simulink model "WDS_MHE"  (R2022a)
settings: Solver=FixedStepDiscrete  StartTime=0.0  StopTime=T_final  FixedStep=T_sample  RelTol=1e-3
values from neighbouring files (symbols this model uses):
  A1 = inv(S1)*IO*U_i.'    [Run_model.m]
  A2 = OI*U_i.'    [Run_model.m]
  A_bar_d = readmatrix('A_bar_d.csv')    [Run_model.m]    (also in prepare_trajectory_data.m = [0.9950 0.0998)
  A_in1 = [zeros(size(HL_u,1),T*n_states), HL_u ... (first row only)    [Run_model.m]
  A_in2 = [zeros(size(HL_u,1),n_meas*T) ... (first row only)    [Run_model.m]
  b1p = inv(S1)*IO*U_history.'    [Run_model.m]
  b2p = OI*U_history.'    [Run_model.m]
  B_bar_d = readmatrix('B_bar_d.csv')    [Run_model.m]    (also in prepare_trajectory_data.m = [0.1)
  BDD_thresh = 5    [Run_model.m]
  C_obsv_d = [-0.48244804282  -0.463279461508; 0.0144227342104  -0.230554726046; 0.244765695792  -0.329721244669; 0.487562807757  0.730038636795; 0.684075320502  -0.191202440855; 0.0380669049625  0.232348391545]    [C_obsv_d.mat]    (also in Run_model.m = readmatrix('C_obsv_d.csv'); sys_generation_WDS.m = C_obsv)
  CE_MH = kron(eye(T),C_E)    [Run_model.m]
  Cm = ones(1,n_states)    [Run_model.m]
  D_obsv_d = readmatrix('D_obsv_d.csv')    [Run_model.m]    (also in prepare_trajectory_data.m = zeros(n_meas,n_int); sys_generation_WDS.m = D_obsv)
  DE_MH = kron(eye(T),D_E)    [Run_model.m]
  e_ini_matrix = reshape(e_ini,n_meas,T)    [Run_model.m]
  E_MH = kron(eye(T),E)    [Run_model.m]
  I = sort(randperm(n_meas,n_attack)).'    [Run_model.m]
  I_attack_ini = repmat(I,1,T)    [Run_model.m]
  K = place(A_bar_d,B_bar_d,Pc)    [Run_model.m]
  max_iter = 5000    [Run_model.m]
  n_alpha = size(HL_u,2)    [Run_model.m]
  n_meas = size(C_obsv_d,1)    [Run_model.m]    (also in prepare_trajectory_data.m = 6; sys_generation_WDS.m = size(C_obsv,1); test.m = size(C,1))
  n_states = 10    [sys_generation_WDS.m]    (also in test.m = size(A,1))
  offset = -inv(B_bar_d)*(A_bar_d-eye(n_states))*xd    [Run_model.m]
  T = 2*n_states    [Run_model.m]    (also in prepare_trajectory_data.m = 5)
  T_sample = 0.01    [Run_model.m]    (also in plot_error_table.m; prepare_trajectory_data.m; sys_generation_WDS.m; test.m)
  T_start_attack = .2*T_final    (= 1.6)    [Run_model.m]
  T_start_opt = load('Results/Data3.mat').T_start_opt    [plot_error_table.m]
  U0 = zeros(n_int,T+1)    [Run_model.m]
  x0 = 0.3+ 0.2*rand(n_states,1)    [Run_model.m]    (also in prepare_trajectory_data.m = [7;7]; test.m = rand(n_states,1))
  xd = 0.5*ones(n_states,1)    [Run_model.m]
  Y0 = zeros(n_meas,T)    [Run_model.m]
libraries: simulink x3
settings Model: Creator=Abelb  LastModifiedBy=Abelb
settings DebuggingCC: UnconnectedInputMsg=warning  UnconnectedOutputMsg=warning  UnconnectedLineMsg=warning
settings RTWCC: DLArmComputeVersion=19.05

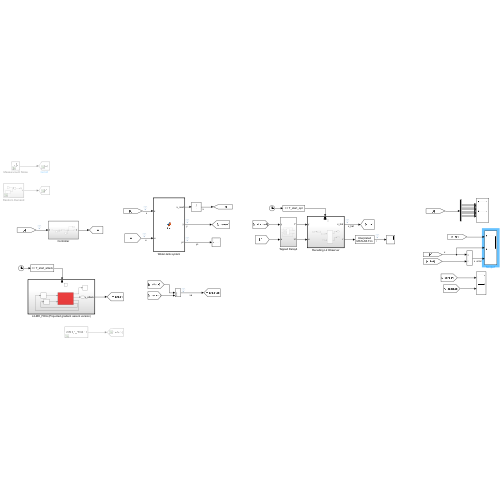
[thumbnail: Simulink's stored preview of the top-level diagram]
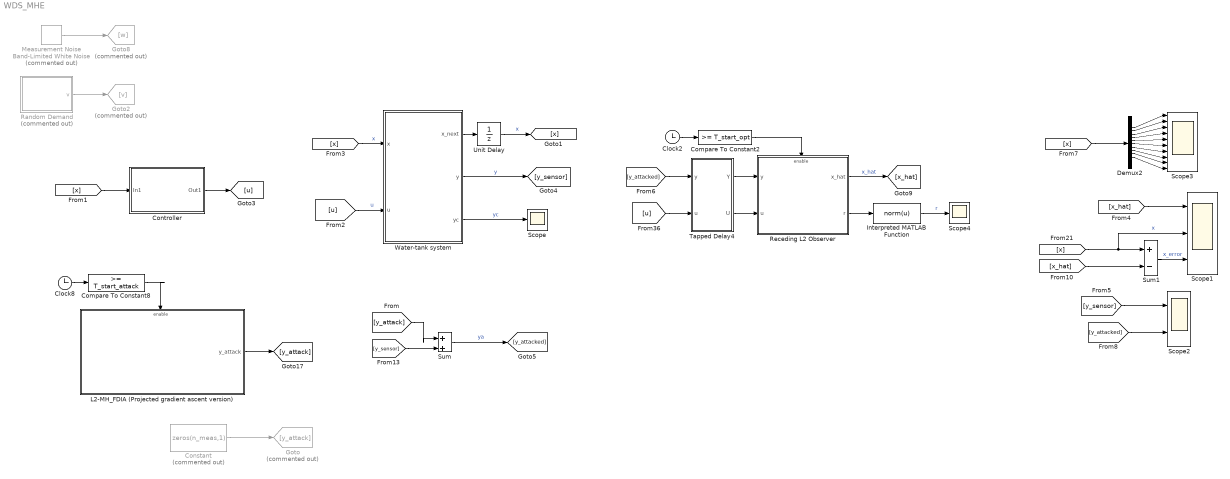
== system WDS_MHE ==
  Clock2 : Clock
  Clock8 : Clock
  Compare To Constant2 : simulink/Logic and Bit Operations/Compare To Constant  relop=>=  const=T_start_opt  OutDataTypeStr=boolean
  Compare To Constant8 : simulink/Logic and Bit Operations/Compare To Constant  relop=>=  const=T_start_attack  OutDataTypeStr=boolean
  Constant : Constant  Commented=on  Value=zeros(n_meas,1)
  Controller : Subsystem
  Demux2 : Demux  Outputs=n_states
  Goto : Goto  Commented=on  GotoTag=y_attack
  Goto2 : Goto  Commented=on  GotoTag=v
  Goto8 : Goto  Commented=on  GotoTag=w
  Interpreted MATLAB Function : MATLABFcn  MATLABFcn=norm(u)
  L2-MH_FDIA (Projected gradient ascent version) : Subsystem
  Measurement Noise : simulink/Sources/Band-Limited White Noise  Commented=on  Cov=[0.001]  Ts=T_sample  seed=[23341]
  Random Demand : Subsystem  Commented=on
  Receding L2 Observer : Subsystem
  Scope : Scope
  Scope1 : Scope  NumInputPorts=3
  Scope2 : Scope  NumInputPorts=2
  Scope3 : Scope  NumInputPorts=10
  Scope4 : Scope
  Sum : Sum  Inputs=|++
  Sum1 : Sum  Inputs=+-
  Tapped Delay4 : Subsystem
  Unit Delay : UnitDelay  InitialCondition=x0  SampleTime=-1  HasFrameUpgradeWarning=on
  Water-tank system : MATLAB Function  TreatAsAtomicUnit=on
  wires:
  Water-tank system/1(x_next) -> Unit Delay/1
  [u] -> Water-tank system/2(u)  "u"
  Tapped Delay4/2(U) -> Receding L2 Observer/2(u)
  Receding L2 Observer/1(x_hat) -> [x_hat]  "x_hat"
  [u] -> Tapped Delay4/2(u)
  Compare To Constant2/1 -> Receding L2 Observer/Enable
  Tapped Delay4/1(Y) -> Receding L2 Observer/1(y)
  Clock2/1 -> Compare To Constant2/1
  Demux2/4 -> Scope3/4
  Demux2/3 -> Scope3/3
  Demux2/5 -> Scope3/5
  Demux2/9 -> Scope3/9
  Demux2/10 -> Scope3/10
  Demux2/7 -> Scope3/7
  Demux2/1 -> Scope3/1
  Demux2/6 -> Scope3/6
  Demux2/2 -> Scope3/2
  Demux2/8 -> Scope3/8
  Interpreted MATLAB Function/1 -> Scope4/1  "r"
  Receding L2 Observer/2(r) -> Interpreted MATLAB Function/1
  [x] -> Controller/1(In1)
  Controller/1(Out1) -> [u]
  [x] -> Demux2/1
  Sum1/1 -> Scope1/3  "x_error"
  [x] -> Scope1/2, Sum1/1  "x"
  [x_hat] -> Sum1/2
  Water-tank system/3(yc) -> Scope/1  "yc"
  Unit Delay/1 -> [x]  "x"
  [x] -> Water-tank system/1(x)  "x"
  [x_hat] -> Scope1/1
  Compare To Constant8/1 -> L2-MH_FDIA (Projected gradient ascent version)/Enable
  Clock8/1 -> Compare To Constant8/1
  L2-MH_FDIA (Projected gradient ascent version)/1(y_attack) -> [y_attack]
  [y_sensor] -> Scope2/1
  [y_attacked] -> Tapped Delay4/1(y)
  Constant/1 -> Goto/1
  Measurement Noise/1 -> Goto8/1
  Random Demand/1(v) -> Goto2/1
  Water-tank system/2(y) -> [y_sensor]  "y"
  [y_sensor] -> Sum/2
  [y_attack] -> Sum/1
  Sum/1 -> [y_attacked]  "ya"
  [y_attacked] -> Scope2/2

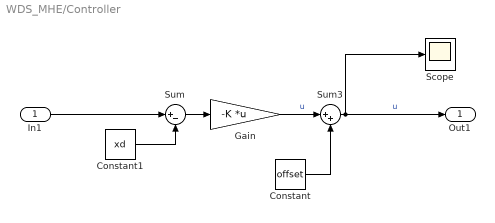
== system WDS_MHE/Controller ==
  In1 : Inport
  Constant : Constant  Value=offset
  Constant1 : Constant  Value=xd
  Gain : Gain  Gain=-K  Multiplication=Matrix(K*u) (u vector)
  Scope : Scope
  Sum : Sum  Inputs=|+-
  Sum3 : Sum  Inputs=|++
  Out1 : Outport
  wires:
  Sum3/1 -> Out1/1, Scope/1  "u"
  Constant/1 -> Sum3/2
  Constant1/1 -> Sum/2
  Sum/1 -> Gain/1
  In1/1 -> Sum/1
  Gain/1 -> Sum3/1  "u"

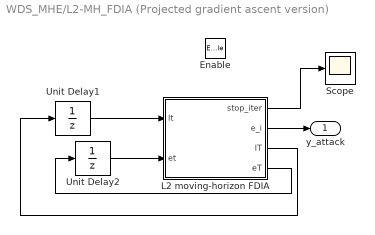
== system WDS_MHE/L2-MH_FDIA (Projected gradient ascent version) ==
  Enable : EnablePort
  L2 moving-horizon FDIA : MATLAB Function  TreatAsAtomicUnit=on
  Scope : Scope
  Unit Delay1 : UnitDelay  InitialCondition=I_attack_ini  SampleTime=-1  HasFrameUpgradeWarning=on
  Unit Delay2 : UnitDelay  InitialCondition=e_ini_matrix  SampleTime=-1  HasFrameUpgradeWarning=on
  y_attack : Outport
  wires:
  L2 moving-horizon FDIA/2(e_i) -> y_attack/1
  Unit Delay1/1 -> L2 moving-horizon FDIA/1(It)
  Unit Delay2/1 -> L2 moving-horizon FDIA/2(et)
  L2 moving-horizon FDIA/3(IT) -> Unit Delay1/1
  L2 moving-horizon FDIA/4(eT) -> Unit Delay2/1
  L2 moving-horizon FDIA/1(stop_iter) -> Scope/1

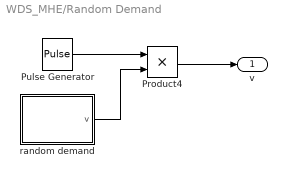
== system WDS_MHE/Random Demand ==
  " random demand" : MATLAB Function  TreatAsAtomicUnit=on
  Product4 : Product
  Pulse Generator : DiscretePulseGenerator  Period=10  SampleTime=T_sample
  v : Outport
  wires:
  " random demand"/1(v) -> Product4/2
  Product4/1 -> v/1
  Pulse Generator/1 -> Product4/1

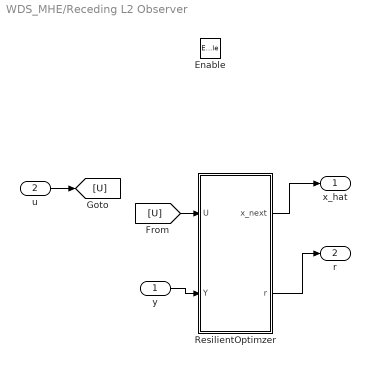
== system WDS_MHE/Receding L2 Observer ==
  y : Inport
  u : Inport  Port=2
  Enable : EnablePort
  ResilientOptimzer : MATLAB Function  TreatAsAtomicUnit=on
  x_hat : Outport
  r : Outport  Port=2
  wires:
  u/1 -> [U]
  y/1 -> ResilientOptimzer/2(Y)
  [U] -> ResilientOptimzer/1(U)
  ResilientOptimzer/1(x_next) -> x_hat/1
  ResilientOptimzer/2(r) -> r/1

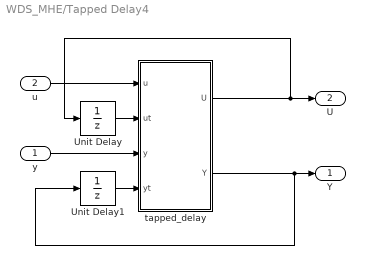
== system WDS_MHE/Tapped Delay4 ==
  y : Inport
  u : Inport  Port=2
  Unit Delay : UnitDelay  InitialCondition=U0  SampleTime=-1  HasFrameUpgradeWarning=on
  Unit Delay1 : UnitDelay  InitialCondition=Y0  SampleTime=-1  HasFrameUpgradeWarning=on
  tapped_delay : MATLAB Function  TreatAsAtomicUnit=on
  Y : Outport
  U : Outport  Port=2
  wires:
  u/1 -> tapped_delay/1(u)
  y/1 -> tapped_delay/3(y)
  tapped_delay/1(U) -> Unit Delay/1, U/1
  tapped_delay/2(Y) -> Unit Delay1/1, Y/1
  Unit Delay/1 -> tapped_delay/2(ut)
  Unit Delay1/1 -> tapped_delay/4(yt)

== matlab function WDS_MHE/Random Demand/ random demand ==
  data: v output; n_states parameter
function v = fcn(n_states)

v = 0.3*rand(n_states,1);

== matlab function WDS_MHE/Water-tank system ==
  data: x input; x_next output; u input; y output; A_bar_d parameter; C_obsv_d parameter; B_bar_d parameter; D_obsv_d parameter; Cm parameter; yc output
function [x_next,y,yc] = fcn(x,u,A_bar_d,C_obsv_d,B_bar_d,D_obsv_d,Cm)
% Discrete state-space model for system

x_next = A_bar_d*x + B_bar_d*u;

y = C_obsv_d*x + D_obsv_d*u;

% critical measurements
yc = Cm*x;

== matlab function WDS_MHE/Tapped Delay4/tapped_delay ==
  data: u input; U output; ut input; y input; yt input; Y output
function [U,Y] = fcn(u,ut,y,yt)
%% tapped_delay_array
% shift columns from tapped matrix to the left and appends most recent
% vector to the last column
%%% input
ut(:,1:end-1) = ut(:,2:end);
ut(:,end) = u;
U = ut;
%%% output
yt(:,1:end-1) = yt(:,2:end);
yt(:,end) = y;
Y = yt;

== matlab function WDS_MHE/Receding L2 Observer/ResilientOptimzer ==
  data: x_next output; U input; Y input; A_in1 parameter; A_in2 parameter; n_states parameter; E_MH parameter; T parameter; r output; CE_MH parameter; n_alpha parameter; DE_MH parameter
% function [x_next,r]  = fcn(U,Y, Ly, Lu,H0_perp, H1)                                 % MD L2  
% function [x_next,r]  = fcn(U,Y,T, H0,H1,F,A_bar_d,n_states)                            % MD L1
% function [x_next,r]  = fcn(U,Y, Aeq,n_states,E_MH,T, CE_MH, n_alpha, DE_MH)          % DD L2, DD L1
function [x_next,r]  = fcn(U,Y, A_in1,A_in2, n_states,E_MH,T, CE_MH, n_alpha, DE_MH)    % DD L1

%% MD L2
%% function [x_next,r]  = fcn(U,Y, Ly, Lu,H0_perp, H1)   
% % vectorized
% u_local = U(:,1:end-1);
% u = u_local(:);
% y = Y(:);
% 
% x_next = zeros(10,1);
% r = zeros(size(y,1),1);
% 
% x_next(:) = Ly*y + Lu*u;
% r(:) = H0_perp*(y-H1*u);


%% DD L2
%% function [x_next,r]  = fcn(U,Y, Aeq,n_states,E_MH,T, DE_MH, n_alpha, CE_MH)
% % vectorized
% u_local = U(:,2:end);
% u = u_local(:);
% y = Y(:);
% 
% x_next = zeros(10,1);
% r = zeros(size(y,1),1);
% 
% coder.extrinsic('DD_L2_MHE');
% [x_next(:)] = DD_L2_MHE(y,u,T,Aeq,n_states,E_MH,CE_MH,DE_MH,n_alpha);


%% MD L1
%% function [x_next,r]  = fcn(U,Y,T, H0,H1,F,A_bar_d,n_states) 
% % vectorized
% u_local = U(:,1:end-1);
% u = u_local(:);
% y = Y(:);
% 
% x_next = zeros(10,1);
% r = zeros(size(y,1),1);
% 
% coder.extrinsic('L1_MHE');
% [x_next(:),r(:)] = L1_MHE(y,u,T,H0,H1,F,A_bar_d,n_states);


%% DD L1
%% function [x_next,r]  = fcn(U,Y, Aeq,n_states,E_MH,T, DE_MH, n_alpha, CE_MH)
% vectorized
u_local = U(:,2:end);
u = u_local(:);
y = Y(:);

x_next = zeros(10,1);
r = zeros(size(y,1),1);

coder.extrinsic('DD_L1_MHE');
[x_next(:)] = DD_L1_MHE(y,u,T,A_in1, A_in2,n_states,E_MH,CE_MH,DE_MH,n_alpha);

== matlab function WDS_MHE/L2-MH_FDIA (Projected gradient ascent version)/L2 moving-horizon FDIA ==
  data: stop_iter output; A1 parameter; BDD_thresh parameter; It input; et input; T parameter; n_meas parameter; A2 parameter; b1p parameter; b2p parameter; e_i output; IT output; eT output; max_iter parameter; I parameter
function [stop_iter,e_i,IT,eT] = fcn(A1,BDD_thresh,It,et, T, n_meas, A2, b1p, b2p,max_iter,I)
%% generate moving-horizon attack

%% unpacking inputs
et_temp = et(:,2:end);
e_history = et_temp;

It_temp = It(:,2:end);
I_history = It_temp;


%% solve the current attack
I_i = I;  % attack support

[stop_iter,e_i] = L2_MH_FDIA(A1,A2,b1p,b2p,I_history,e_history,I_i,T,n_meas,T*BDD_thresh,max_iter);

% eps0 = norm(A2*e_i+b2p*e_history(:));
% eps2 = norm(G2*[et(:);e_i]);
%% store the attack vectors and supports
et(:,1:end-1) = et(:,2:end);
et(:,end) = e_i;
eT = et;
% 
% eps1 = norm(G1*eT(:));


It(:,1:end-1) = It(:,2:end);
It(:,end) = I_i;
IT = It;
